simulink model "ProjectSimulationv1"  (R2020a)
settings: Solver=FixedStepDiscrete  StartTime=0.0  StopTime=2  RelTol=1e-3
undefined symbols (not defined in the file): Acid, Down, Lead, Up
libraries: powerlib x36, eeGeneralControl x4, electricdrivelib x1, simulink x1, eePwmGenerator x1
settings Model: Creator=Asus  LastModifiedBy=asus
settings DataIOCC: ReturnWorkspaceOutputs=off
settings DebuggingCC: ArithmeticOperatorsInVariantConditions=warning
settings SFSimCC: CustomCodeUndefinedFunction=UseInterfaceOnly

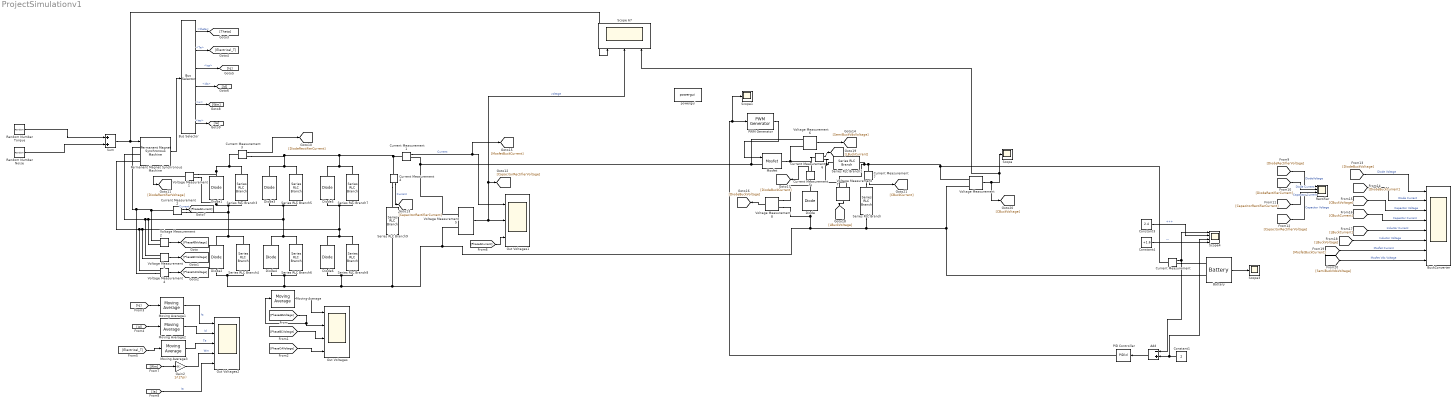
== system ProjectSimulationv1 ==
  Add : Sum  Inputs=-+
  Battery : electricdrivelib/Extra Sources/Battery  BatType=Lead-Acid  ShowTempParam=off  ThermalPreset=no  ShowAgeParam=off  NomV=24  NomQ=13  SOC=50  Batt_Tr=0.000001  PresetModel=on  MaxQ=13.5417  MinV=18  FullV=26.1316  Dis_rate=2.6  R=0.018462  Normal_OP=4.0336  expZone="[24.4342    0.0433333]"  current=[6.5 13 32.5]  Units=Time  Tci=20  NomT=20  T2=-30  MaxQ2=4.8  FullV2=7.1  Normal_OP2=5.655  expZone2="[6.58           1]"  Rca=0.6  ti=2000  Dp=0  Neq0=0  Tsim=1e6  Ta1=25  Qeol=5.4*0.9  Reol=0.013333*1.2  Char_age=[2.3478, 3]  Dis_age=[2.3478, 10]  N1=1500  N2=10500  N3=1000  N4=1400  Ta2=45  N5=950
  BuckConverter : Scope  NumInputPorts=8
  Bus Selector : BusSelector  OutputSignals=theta,Te,iqs,ids,w,ias
  Constant1 : Constant  Value=2
  Constant3 : Constant  Value=2.4
  Constant4 : Constant  Value=+1.6
  Current Measurement{,1..7} (8 alike) : powerlib/Measurements/Current Measurement  PhasorSimulation=off  OutputType=Complex  PSBequivalent=0
  Diode : powerlib/Power Electronics/Diode  Ron=0.05  Lon=0  Vf=1.25  IC=0  UseSnubber=0  Rs=1e6  Cs=250e-9  Measurements=off
  Diode{1..6} (6 alike) : powerlib/Power Electronics/Diode  Ron=0.08  Lon=0  Vf=0.9  IC=0  UseSnubber=0  Rs=0  Cs=0  Measurements=off
  Gain2 : Gain  Gain=1/(2*pi)
  Mosfet : powerlib/Power Electronics/Mosfet  Ron=0.95  Lon=0  Rd=1.6667  Vfd=0.85  IC=0  Rs=1e5  Cs=inf  Measurements=off
  Moving Average : eeGeneralControl/Moving Average  VariantControl=Variant1  LabelModeActiveChoice=Discrete  f=1000  x0=0  Ts=10e-6
      settings: SourceProductBaseCode=PS
  Moving Average1 : eeGeneralControl/Moving Average  VariantControl=Variant1  LabelModeActiveChoice=Discrete  f=100  x0=0  Ts=1e-5
      settings: SourceProductBaseCode=PS
  Moving Average2 : eeGeneralControl/Moving Average  VariantControl=Variant1  LabelModeActiveChoice=Discrete  f=100  x0=0  Ts=1e-5
      settings: SourceProductBaseCode=PS
  Moving Average3 : eeGeneralControl/Moving Average  VariantControl=Variant1  LabelModeActiveChoice=Discrete  f=100  x0=0  Ts=1e-5
      settings: SourceProductBaseCode=PS
  Out Voltages : Scope  NumInputPorts=4
  Out Voltages1 : Scope  NumInputPorts=3
  Out Voltages2 : Scope  NumInputPorts=5
  PID Controller : simulink/Continuous/PID Controller  Controller=PID  Form=Parallel  TimeDomain=Discrete-time  UseExternalTs=off  SampleTime=1e-6  IntegratorMethod=Forward Euler  FilterMethod=Forward Euler  ControllerParametersSource=internal  P=25  I=60  D=0  UseFilter=off  N=100  TunerSelectOption=Transfer Function Based (PID Tuner App)  ZeroCross=off  InitialConditionSource=internal  InitialConditionForIntegrator=0  InitialConditionForFilter=0  DifferentiatorICPrevScaledInput=0  ExternalReset=none  TrackingMode=off  Kt=1  LimitOutput=off  UpperSaturationLimit=inf  LowerSaturationLimit=-inf  LinearizeAsGain=on  AntiWindupMode=none  Kb=1  POutMin=[]  POutMax=[]  IOutMin=[]  IOutMax=[]  DOutMin=[]  DOutMax=[]  NOutMin=[]  NOutMax=[]  SumOutMin=[]  SumOutMax=[]  SaturationOutMin=[]  SaturationOutMax=[]  PParamMin=[]  PParamMax=[]  IParamMin=[]  IParamMax=[]  DParamMin=[]  DParamMax=[]  NParamMin=[]  NParamMax=[]  KbParamMin=[]  KbParamMax=[]  KtParamMin=[]  KtParamMax=[]  KbOutMin=[]  KbOutMax=[]  KtOutMin=[]  KtOutMax=[]  IntegratorOutMin=[]  IntegratorOutMax=[]  FilterOutMin=[]  FilterOutMax=[]  SumI1OutMin=[]  SumI1OutMax=[]  SumI2OutMin=[]  SumI2OutMax=[]  SumI3OutMin=[]  SumI3OutMax=[]  SumI4OutMin=[]  SumI4OutMax=[]  SumDOutMin=[]  SumDOutMax=[]  DifferentiatorOutMin=[]  DifferentiatorOutMax=[]  FilterDiffOutCoefMin=[]  FilterDiffOutCoefMax=[]  ReciprocalOutMin=[]  ReciprocalOutMax=[]  SumDenOutMin=[]  SumDenOutMax=[]  SumNumOutMin=[]  SumNumOutMax=[]  DivideOutMin=[]  DivideOutMax=[]  UdiffTsProdOutMin=[]  UdiffTsProdOutMax=[]  NTsProdOutMin=[]  NTsProdOutMax=[]  UintegralTsProdOutMin=[]  UintegralTsProdOutMax=[]  UngainTsProdOutMin=[]  UngainTsProdOutMax=[]  IntegratorContinuousStateAttributes=''  IntegratorStateMustResolveToSignalObject=off  IntegratorRTWStateStorageClass=Auto  FilterContinuousStateAttributes=''  FilterStateMustResolveToSignalObject=off  FilterRTWStateStorageClass=Auto  ParallelPVariant=InternalParameters  IdealPVariant=Disabled  IVariant=InternalParameters  DVariant=InternalParameters  IntegratorVariant=Discrete  SatVariant=Disabled  AWVariant=Passthrough  PCopyVariant=Disabled  TRVariant=Disabled  FdbkBlocksVariant=Forward  IdealPFdbkVariant=Disabled  SatFdbkVariant=Disabled  DerivativeFilterVariant=Differentiator  NVariant=Passthrough  NCopyVariant=Disabled_SignalSpec  FilterICVariant=InternalICsDifferentiator  IntegratorICVariant=InternalICs  ExternalResetVariant=Disabled  TRSumVariant=Passthrough  SumFdbkVariant=Disabled  SumVariant=Sum_PID  TsampFilterVariant=InternalTs  TsampNgainVariant=Passthrough  TsampIntegralVariant=Passthrough
  PWM Generator : eePwmGenerator/PWM Generator  CarrCount=Up-Down  Tper=2e-5  Ts=1e-6
  Permanent Magnet Synchronous Machine : powerlib/Machines/Permanent Magnet Synchronous Machine  NbPhases=3  FluxDistribution=Sinusoidal  RotorType=Round  MechanicalLoad=Torque Tm  PresetModel=No  ShowDetailedParameters=on  MeasurementBus=on  Resistance=10.58  Inductance=8.5e-3  dqInductances=[8.5e-3,8.5e-3]  La=16.7e-3  MachineConstant=Voltage Constant (V_peak L-L / krpm)  Flux=0.60646  VoltageCst=110  TorqueCst=0.90969  Flat=120  Mechanical=[0.00027 0.005024 1 0]  PolePairs=4  InitialConditions=[100,0, 0,0]  InitialConditions5ph=[0 0 0 0 0 0]  RefAngle=90 degrees behind phase A axis (modified Park)  IterativeDiscreteModel=Trapezoidal non iterative  TsBlock=-1  TsPowergui=0
  Random Number Noise : RandomNumber  Variance=0.1  SampleTime=1e-3
  Random Number Torque : RandomNumber  Mean=-1.6  Variance=0.05  SampleTime=0.1
  Rectifier : Scope  NumInputPorts=4
  Scope : Scope
  Scope 67 : Scope  NumInputPorts=3
  Scope1 : Scope
  Scope3 : Scope
  Scope4 : Scope  NumInputPorts=4
  Series RLC Branch : powerlib/Elements/Series RLC Branch  LConnTagsString=__new0  RConnTagsString=__new0  BranchType=RC  Resistance=0.22  Inductance=1e-9  SetiL0=off  InitialCurrent=0  Capacitance=68e-6  Setx0=on  InitialVoltage=24.1  Measurements=None
  Series RLC Branch1 : powerlib/Elements/Series RLC Branch  LConnTagsString=__new0  RConnTagsString=__new0  BranchType=L  Resistance=1  Inductance=0.012  SetiL0=off  InitialCurrent=0  Capacitance=1e-6  Setx0=off  InitialVoltage=0  Measurements=None
  Series RLC Branch{3..8} (6 alike) : powerlib/Elements/Series RLC Branch  LConnTagsString=__new0  RConnTagsString=__new0  BranchType=R  Resistance=1e6  Inductance=1e-3  SetiL0=off  InitialCurrent=0  Capacitance=1e-6  Setx0=off  InitialVoltage=0  Measurements=None
  Series RLC Branch9 : powerlib/Elements/Series RLC Branch  LConnTagsString=__new0  RConnTagsString=__new0  BranchType=C  Resistance=1e6  Inductance=1e-3  SetiL0=off  InitialCurrent=0  Capacitance=56e-6  Setx0=on  InitialVoltage=225  Measurements=None
  Sum : Sum  Inputs=+|+
  Voltage Measurement{,1..8} (9 alike) : powerlib/Measurements/Voltage Measurement  PhasorSimulation=off  OutputType=Complex  PSBequivalent=0
  powergui : powerlib/powergui  Priority=1  SimulationMode=Discrete  SampleTime=1e-7  frequency=60  Iterations=50  frequencyindice=0  Pbase=100e6  ErrMax=1e-4  UnitsV=kV  UnitsW=MW  buscounter=0  FunctionMessages=off  echomessages=off  EnableUseOfTLC=off  CurrentSourceSwitches=off  DisableSnubberDevices=off  DisableRonSwitches=off  DisableVfSwitches=off  DisplayEquations=off  AutomaticDiscreteSolvers=off  SolverType=Tustin/Backward Euler (TBE)  Interpol=off  ExternalGateDelay=off  methode=off  Ts=100  x0status=blocks  SPID=on  SwTol=0  HookPort=off  NonlinearTolerance=1e-4  nMaxIteration=100  ContinueOnMaxIteration=off  RestoreLinks=warning  ResistiveCurrentMeasurement=off  Frange=[0:2:500]  Ylog=off  Xlog=on  ShowGrid=off  save=off  variable=ZData  structure=0  ZoomFFT=off  StartTime=0.0  cycles=1  DisplayStyle=1  fundamental=60  FreqAxis=off  MaxFrequency=1000  frequencyindicesteady=1  RmsSteady=1  display=off
  wires:
  PWM Generator/1 -> Mosfet/1
  Voltage Measurement/1 -> [CBuckVoltage], Scope 67/3, Scope/1
  Constant3/1 -> Scope4/2  "+++"
  Current Measurement/1 -> Scope4/1, Add/1
  Add/1 -> PID Controller/1
  Constant1/1 -> Scope4/3, Add/2
  Constant4/1 -> Scope4/4  "---"
  Battery/1 -> Scope3/1
  Moving Average1/1 -> Out Voltages2/1  "Iq"
  Bus Selector/4 -> [Id]  "<ids>"
  [Ia] -> Out Voltages2/5  "Ia"
  Bus Selector/6 -> [Ia]  "<ias>"
  Bus Selector/5 -> [Wm]  "<w>"
  [Wm] -> Gain2/1
  [PhaseACurrent] -> Out Voltages1/3
  [Electrical_T] -> Moving Average3/1
  Current Measurement2/1 -> [PhaseACurrent]  "Current"
  Moving Average2/1 -> Out Voltages2/2  "Id"
  [PhaseCAVoltage] -> Out Voltages/4
  Bus Selector/3 -> [Iq]  "<iqs>"
  [Id] -> Moving Average2/1
  [Iq] -> Moving Average1/1
  Permanent Magnet Synchronous Machine/1 -> Bus Selector/1
  [PhaseABVoltage] -> Moving Average/1, Out Voltages/2
  Voltage Measurement3/1 -> [PhaseBCVoltage]
  Voltage Measurement2/1 -> [PhaseABVoltage]
  Random Number Torque/1 -> Sum/1
  Bus Selector/1 -> [Theta]  "<theta>"
  Current Measurement1/1 -> [MosfetBuckCurrent], Out Voltages1/1  "Current"
  Voltage Measurement4/1 -> [PhaseCAVoltage]
  Random Number Noise/1 -> Sum/2
  Voltage Measurement5/1 -> Scope 67/2, [CapacitorRectifierVoltage], Out Voltages1/2  "voltage"
  Gain2/1 -> Out Voltages2/4  "Wm"
  Bus Selector/2 -> [Electrical_T]  "<Te>"
  Moving Average3/1 -> Out Voltages2/3  "Te"
  Moving Average/1 -> Out Voltages/1
  [PhaseBCVoltage] -> Out Voltages/3
  Sum/1 -> Scope 67/1, Permanent Magnet Synchronous Machine/1
  Current Measurement3/1 -> [DiodeRectifierCurrent]
  Voltage Measurement1/1 -> [DiodeRectifierVoltage]
  Current Measurement4/1 -> [CapacitorRectifierCurrent]  "Current"
  Voltage Measurement6/1 -> [SemiBuckVdsVoltage]
  Voltage Measurement8/1 -> [DiodeBuckVoltage]
  Current Measurement5/1 -> [DiodeBuckCurrent]
  Voltage Measurement7/1 -> [LBuckVoltage]
  Current Measurement6/1 -> [LBuckCurrent]
  Current Measurement7/1 -> [CBuckCurrent]
  [DiodeRectifierVoltage] -> Rectifier/1  "DiodeVoltage"
  [DiodeRectifierCurrent] -> Rectifier/2  "Diode Current"
  [CapacitorRectifierCurrent] -> Rectifier/3  "Capacitor Current"
  [CapacitorRectifierVoltage] -> Rectifier/4  "Capacitor Voltage"
  [DiodeBuckVoltage] -> BuckConverter/1  "Diode Voltage"
  [DiodeBuckCurrent] -> BuckConverter/2  "Diode Current"
  [CBuckVoltage] -> BuckConverter/3  "Capacitor Voltage"
  [CBuckCurrent] -> BuckConverter/4  "Capacitor Current"
  [LBuckCurrent] -> BuckConverter/5  "Inductor Current"
  [LBuckVoltage] -> BuckConverter/6  "Inductor Voltage"
  [MosfetBuckCurrent] -> BuckConverter/7  "Mosfet Current"
  [SemiBuckVdsVoltage] -> BuckConverter/8  "Mosfet Vds Voltage"
  PID Controller/1 -> Scope1/1, PWM Generator/1
  connections:
  Current Measurement1/RConn1 -- Voltage Measurement5/LConn1 -- Voltage Measurement6/LConn1 -- Mosfet/LConn1
  Series RLC Branch1/LConn1 -- Voltage Measurement7/LConn1 -- Current Measurement6/RConn1
  Diode4/LConn1 -- Diode2/LConn1 -- Series RLC Branch4/RConn1 -- Diode6/LConn1 -- Series RLC Branch8/RConn1 -- Series RLC Branch9/RConn1 -- Voltage Measurement/LConn2 -- Battery/LConn2 -- Series RLC Branch/RConn1 -- Voltage Measurement8/LConn1 -- Diode/LConn1 -- Voltage Measurement5/LConn2 -- Series RLC Branch6/RConn1
  Voltage Measurement/LConn1 -- Current Measurement/LConn1 -- Current Measurement7/LConn1 -- Voltage Measurement7/LConn2 -- Series RLC Branch1/RConn1
  Current Measurement/RConn1 -- Battery/LConn1
  Diode5/LConn1 -- Series RLC Branch7/RConn1 -- Diode6/RConn1 -- Series RLC Branch8/LConn1 -- Permanent Magnet Synchronous Machine/LConn3 -- Voltage Measurement4/LConn1 -- Voltage Measurement3/LConn2
  Voltage Measurement4/LConn2 -- Current Measurement2/LConn1 -- Voltage Measurement2/LConn1 -- Permanent Magnet Synchronous Machine/LConn1
  Series RLC Branch5/RConn1 -- Series RLC Branch6/LConn1 -- Diode4/RConn1 -- Permanent Magnet Synchronous Machine/LConn2 -- Voltage Measurement3/LConn1 -- Voltage Measurement2/LConn2 -- Diode3/LConn1
  Diode3/RConn1 -- Current Measurement3/RConn1 -- Current Measurement4/LConn1 -- Current Measurement1/LConn1 -- Series RLC Branch7/LConn1 -- Diode5/RConn1 -- Series RLC Branch5/LConn1
  Series RLC Branch3/RConn1 -- Voltage Measurement1/LConn1 -- Diode1/LConn1 -- Current Measurement2/RConn1 -- Series RLC Branch4/LConn1 -- Diode2/RConn1
  Diode1/RConn1 -- Current Measurement3/LConn1 -- Series RLC Branch3/LConn1 -- Voltage Measurement1/LConn2
  Current Measurement4/RConn1 -- Series RLC Branch9/LConn1
  Voltage Measurement8/LConn2 -- Diode/RConn1 -- Current Measurement5/LConn1
  Current Measurement5/RConn1 -- Current Measurement6/LConn1 -- Voltage Measurement6/LConn2 -- Mosfet/RConn1
  Current Measurement7/RConn1 -- Series RLC Branch/LConn1
